simulink model "fast_sim"  (R2018b)
settings: Solver=VariableStepAuto  StartTime=0.0  StopTime=60  RelTol=1e-3
values from neighbouring files (symbols this model uses):
  A = [0 1 0 ... (first row only)    [fast_controller.m]
  B = [0; 0; K/T]    [fast_controller.m]
  C = [1 0 0;0 1 0;0 0 1]    [fast_controller.m]
  K_aw = 0.4    [fast_controller.m]
  Nbar = Nu + K_(2:3)*Nx    [fast_controller.m]
undefined symbols (not defined in the file or in its folder): K_
settings Model: Creator=jasteind  LastModifiedBy=jenny

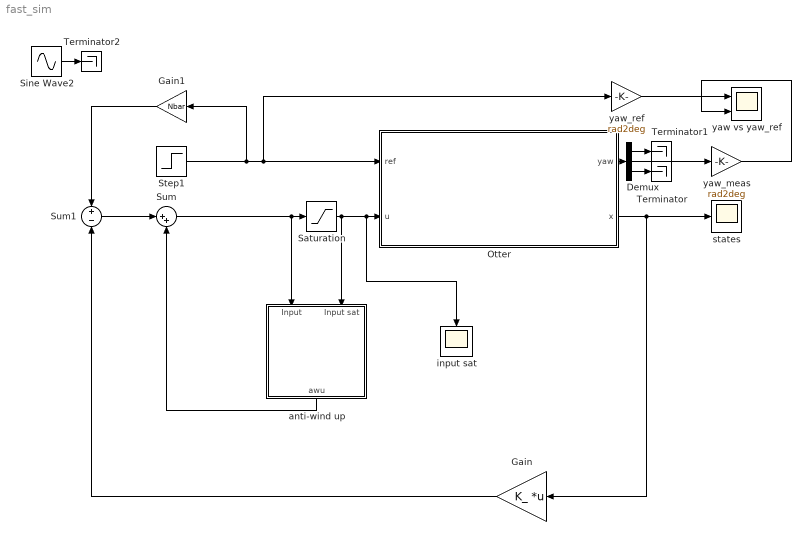
== system fast_sim ==
  Demux : Demux  Outputs=3
  Gain : Gain  Gain=K_  Multiplication=Matrix(K*u)
  Gain1 : Gain  Gain=Nbar
  Otter : Subsystem
  Saturation : Saturate  UpperLimit=73.6  LowerLimit=-73.6
  Sine Wave2 : Sin  Amplitude=pi/6  Frequency=0.05  SampleTime=0
  Step1 : Step  Time=0  After=pi/4  SampleTime=0
  Sum : Sum  Inputs=|++
  Sum1 : Sum  Inputs=+|-
  Terminator : Terminator
  Terminator1 : Terminator
  Terminator2 : Terminator
  anti-wind up : Subsystem
  input sat : Scope
  states : Scope
  yaw vs yaw_ref : Scope  NumInputPorts=2
  yaw_meas : Gain  Gain=rad2deg
  yaw_ref : Gain  Gain=rad2deg
  wires:
  Otter/2(x) -> Gain/1, states/1
  Saturation/1 -> Otter/2(u), input sat/1, anti-wind up/2(Input sat)
  yaw_ref/1 -> yaw vs yaw_ref/1
  yaw_meas/1 -> yaw vs yaw_ref/2
  Gain1/1 -> Sum1/1
  Step1/1 -> Gain1/1, yaw_ref/1, Otter/1(ref)
  Gain/1 -> Sum1/2
  Sum1/1 -> Sum/1
  anti-wind up/1(awu) -> Sum/2
  Sum/1 -> anti-wind up/1(Input), Saturation/1
  Otter/1(yaw) -> Demux/1
  Demux/2 -> yaw_meas/1
  Sine Wave2/1 -> Terminator2/1
  Demux/3 -> Terminator/1
  Demux/1 -> Terminator1/1

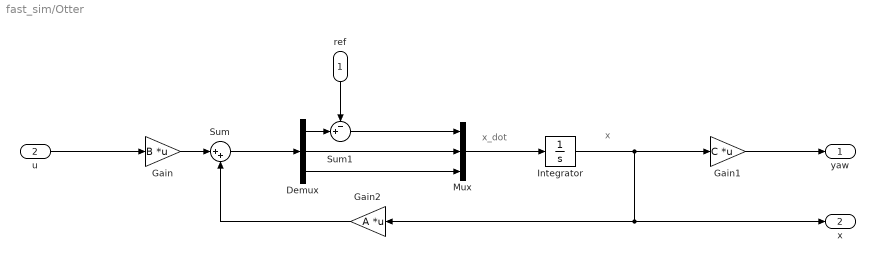
== system fast_sim/Otter ==
  note: x
  note: x_dot
  ref : Inport
  u : Inport  Port=2
  Demux : Demux  Outputs=3
  Gain : Gain  Gain=B  Multiplication=Matrix(K*u)
  Gain1 : Gain  Gain=C  Multiplication=Matrix(K*u)
  Gain2 : Gain  Gain=A  Multiplication=Matrix(K*u)
  Integrator : Integrator
  Mux : Mux  Inputs=3
  Sum : Sum  Inputs=|++
  Sum1 : Sum  Inputs=-+|
  yaw : Outport
  x : Outport  Port=2
  wires:
  Gain/1 -> Sum/1
  Integrator/1 -> Gain1/1, Gain2/1, x/1
  Gain2/1 -> Sum/2
  Gain1/1 -> yaw/1
  Sum/1 -> Demux/1
  Demux/2 -> Mux/2
  Demux/3 -> Mux/3
  Mux/1 -> Integrator/1
  ref/1 -> Sum1/1
  Demux/1 -> Sum1/2
  u/1 -> Gain/1
  Sum1/1 -> Mux/1

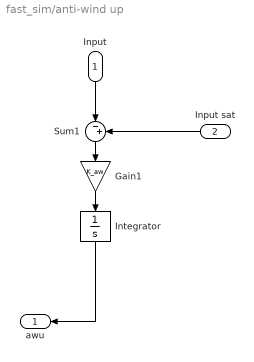
== system fast_sim/anti-wind up ==
  Input : Inport
  Input sat : Inport  Port=2
  Gain1 : Gain  Gain=K_aw
  Integrator : Integrator
  Sum1 : Sum  Inputs=|-+
  awu : Outport
  wires:
  Gain1/1 -> Integrator/1
  Input/1 -> Sum1/1
  Sum1/1 -> Gain1/1
  Input sat/1 -> Sum1/2
  Integrator/1 -> awu/1
